simulink subsystem "Autonomously_Navigate_Poses"  (R2023b)
settings: Solver=VariableStepAuto  StartTime=0.0  StopTime=10.0  RelTol=1e-3
undefined symbols (not defined in the file): Spline_Max_Num_RefPoses, Spline_Num_Samples
settings Model: Creator=FIRSTMentor  LastModifiedBy=FIRSTMentor

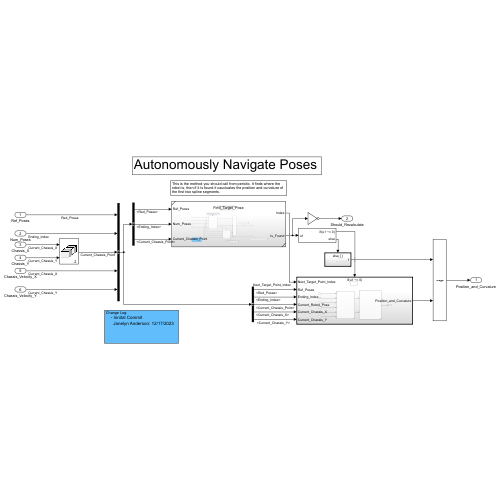
[thumbnail: Simulink's stored preview of the top-level diagram]
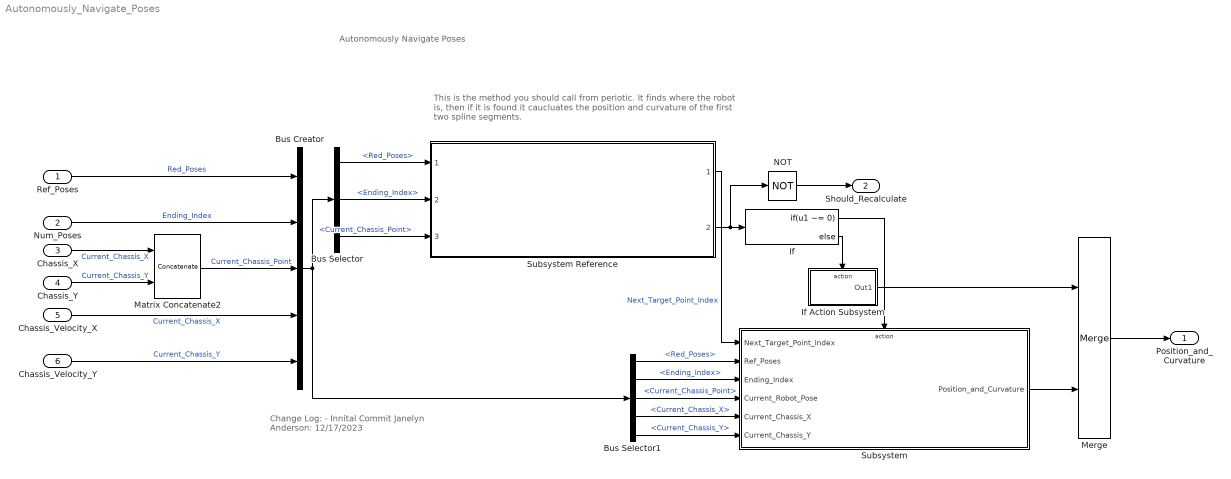
== system Autonomously_Navigate_Poses ==
  note: Autonomously Navigate Poses
  note: This is the method you should call from periotic. It finds where the robot is, then if it is found it caucluates the position and curvature of the first two spline segments.
  note: Change Log:
      | - Innital Commit
      | Janelyn Anderson: 12/17/2023
  Ref_Poses : Inport  OutDataTypeStr=double  PortDimensions=[Spline_Max_Num_RefPoses 2]
  Num_Poses : Inport  Port=2  OutDataTypeStr=int32  Unit=1  PortDimensions=1
  Chassis_X : Inport  Port=3  OutDataTypeStr=double  Unit=m  PortDimensions=1
  Chassis_Y : Inport  Port=4  OutDataTypeStr=double  Unit=m  PortDimensions=1
  Chassis_Velocity_X : Inport  Port=5  OutDataTypeStr=double  Unit=m  PortDimensions=1
  Chassis_Velocity_Y : Inport  Port=6  OutDataTypeStr=double  Unit=m  PortDimensions=1
  Bus Creator : BusCreator  Inputs=5
  Bus Selector : BusSelector  OutputSignals=Red_Poses,Ending_Index,Current_Chassis_Point
  Bus Selector1 : BusSelector  OutputSignals=Red_Poses,Ending_Index,Current_Chassis_Point,Current_Chassis_X,Current_Chassis_Y
  If : If  IfExpression=u1 ~= 0
  If Action Subsystem : Subsystem  TreatAsAtomicUnit=on
  Matrix Concatenate2 : Concatenate  Mode=Multidimensional array  ConcatenateDimension=2
  Merge : Merge
  NOT : Logic  Operator=NOT  IconShape=distinctive  AllPortsSameDT=off  OutDataTypeStr=boolean
  Subsystem : Subsystem
  Subsystem Reference : Subsystem  ReferencedSubsystem=Find_Target_Pose
  Position_and_Curvature : Outport  PortDimensions=[Spline_Num_Samples,3,2]
  Should_Recalculate : Outport  Port=2
  wires:
  If/2 -> If Action Subsystem/Action
  Bus Selector1/3 -> Subsystem/4(Current_Robot_Pose)  "<Current_Chassis_Point>"
  Bus Selector1/5 -> Subsystem/6(Current_Chassis_Y)  "<Current_Chassis_Y>"
  NOT/1 -> Should_Recalculate/1
  Merge/1 -> Position_and_Curvature/1
  Subsystem Reference/2 -> NOT/1, If/1
  If Action Subsystem/1(Out1) -> Merge/1
  Bus Selector1/1 -> Subsystem/2(Ref_Poses)  "<Red_Poses>"
  Bus Selector/3 -> Subsystem Reference/3  "<Current_Chassis_Point>"
  Bus Selector1/2 -> Subsystem/3(Ending_Index)  "<Ending_Index>"
  Bus Creator/1 -> Bus Selector1/1, Bus Selector/1
  Bus Selector1/4 -> Subsystem/5(Current_Chassis_X)  "<Current_Chassis_X>"
  If/1 -> Subsystem/Action
  Bus Selector/1 -> Subsystem Reference/1  "<Red_Poses>"
  Num_Poses/1 -> Bus Creator/2  "Ending_Index"
  Bus Selector/2 -> Subsystem Reference/2  "<Ending_Index>"
  Subsystem/1(Position_and_Curvature) -> Merge/2
  Chassis_Velocity_X/1 -> Bus Creator/4  "Current_Chassis_X"
  Subsystem Reference/1 -> Subsystem/1(Next_Target_Point_Index)  "Next_Target_Point_Index"
  Chassis_Velocity_Y/1 -> Bus Creator/5  "Current_Chassis_Y"
  Ref_Poses/1 -> Bus Creator/1  "Red_Poses"
  Matrix Concatenate2/1 -> Bus Creator/3  "Current_Chassis_Point"
  Chassis_Y/1 -> Matrix Concatenate2/2  "Current_Chassis_Y"
  Chassis_X/1 -> Matrix Concatenate2/1  "Current_Chassis_X"

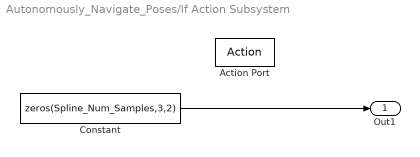
== system Autonomously_Navigate_Poses/If Action Subsystem ==
  Action Port : ActionPort  ActionPortLabel=else
  Constant : Constant  Value=zeros(Spline_Num_Samples,3,2)
  Out1 : Outport
  wires:
  Constant/1 -> Out1/1

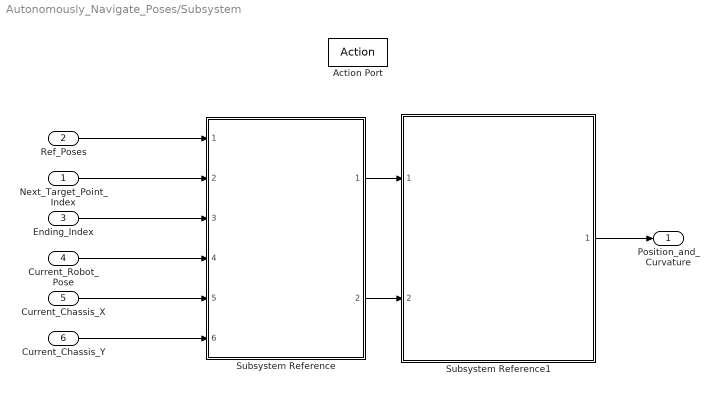
== system Autonomously_Navigate_Poses/Subsystem ==
  Next_Target_Point_Index : Inport
  Ref_Poses : Inport  Port=2
  Ending_Index : Inport  Port=3
  Current_Robot_Pose : Inport  Port=4
  Current_Chassis_X : Inport  Port=5
  Current_Chassis_Y : Inport  Port=6
  Action Port : ActionPort  PropagateVarSize=During execution  ActionPortLabel=if(u1 ~= 0)
  Subsystem Reference : Subsystem  ReferencedSubsystem=Make_Knots
  Subsystem Reference1 : Subsystem  ReferencedSubsystem=Path_Planning
  Position_and_Curvature : Outport  PortDimensions=[Spline_Num_Samples,3,2]
  wires:
  Current_Chassis_Y/1 -> Subsystem Reference/6
  Current_Robot_Pose/1 -> Subsystem Reference/4
  Ref_Poses/1 -> Subsystem Reference/1
  Current_Chassis_X/1 -> Subsystem Reference/5
  Next_Target_Point_Index/1 -> Subsystem Reference/2
  Ending_Index/1 -> Subsystem Reference/3
  Subsystem Reference/1 -> Subsystem Reference1/1
  Subsystem Reference/2 -> Subsystem Reference1/2
  Subsystem Reference1/1 -> Position_and_Curvature/1
